simulink model "modello"  (R2019b)
settings: Solver=ode3  StartTime=0.0  StopTime=Tend  FixedStep=Ts  RelTol=1e-3  EnableMultiTasking=on
undefined symbols (not defined in the file): cart_width, masses, nq, q0, q_cart, qp0, qp_cart, qref0, T, tt, xf, xi, xpf, xpi
settings Model: TunableVars=q0,qp0,qref0  TunableVarsStorageClass=Auto,Auto,Auto  TunableVarsTypeQualifier=,,  Creator=danilo  LastModifiedBy=bhisma
settings DataIOCC: LimitDataPoints=on  SaveFormat=Array  ReturnWorkspaceOutputs=off
settings OptimizationCC: DefaultParameterBehavior=Inlined  LifeSpan=inf
settings DebuggingCC: SolverPrmCheckMsg=warning  SFUnexpectedBacktrackingDiag=warning  SFNoUnconditionalDefaultTransitionDiag=warning  SFExecutionAtInitializationDiag=none  ArithmeticOperatorsInVariantConditions=warning
settings HardwareCC: ProdBitPerPointer=32  ProdBitPerSizeT=32  ProdBitPerPtrDiffT=32  ProdLargestAtomicFloat=None  ProdIntDivRoundTo=Undefined  ProdEndianess=Unspecified  ProdWordSize=32  ProdHWDeviceType=32-bit Generic  TargetBitPerLong=64  TargetBitPerPointer=64  TargetBitPerSizeT=64  TargetBitPerPtrDiffT=64  TargetLongLongMode=on  TargetIntDivRoundTo=Zero  TargetEndianess=LittleEndian  TargetWordSize=64  TargetHWDeviceType=MATLAB Host  ProdEqTarget=off
settings ModelReferenceCC: PropagateSignalLabelsOutOfModel=off
settings SFSimCC: SimUseLocalCustomCode=off  CustomCodeUndefinedFunction=UseInterfaceOnly
settings RTWCC: Description=Rapid Simulation Target  SystemTargetFile=rsim.tlc  TemplateMakefile=rsim_default_tmf  RTWUseLocalCustomCode=off  BuildConfiguration=Faster Runs
settings CodeAppCC: StateflowObjectComments=on  MATLABSourceComments=on
settings RSimTargetCC: PreserveStateflowLocalDataDimensions=off
settings ConfigComp: CovMetricSettings=dw  CovHtmlReporting=on  CovSaveCumulativeToWorkspaceVar=on  CovSaveSingleToWorkspaceVar=on  CovExternalEMLEnable=off  CovSFcnEnable=off

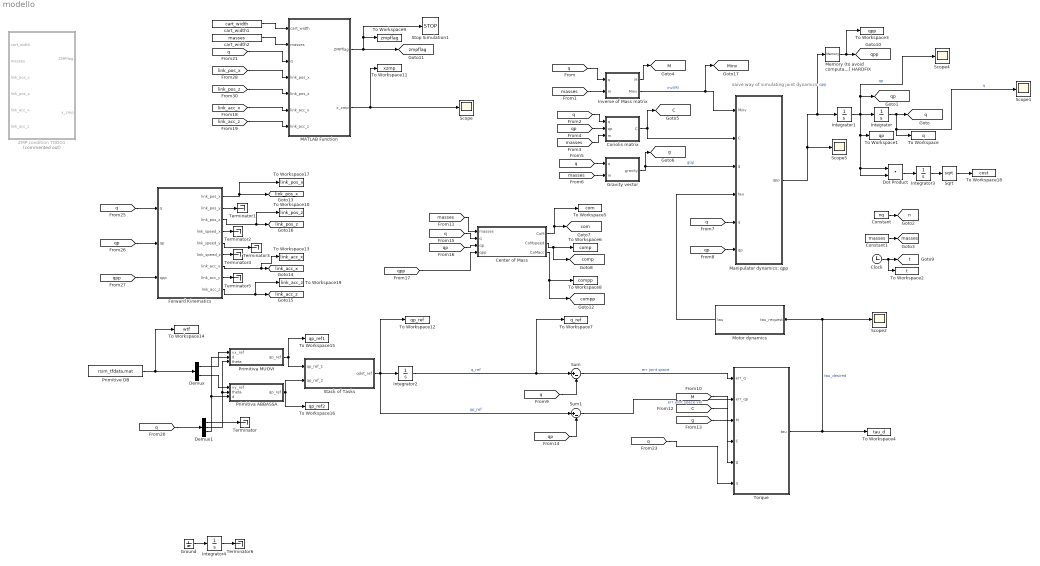
== system modello ==
  note: naive way of simulating joint dynamics
  Center of Mass : MATLAB Function  TreatAsAtomicUnit=on
  Clock : Clock
  Constant : Constant  Value=nq
  Constant1 : Constant  Value=masses
  Coriolis matrix : MATLAB Function  TreatAsAtomicUnit=on
  Demux : Demux  Outputs=2
  Demux1 : Demux  Outputs=3
  Dot Product : DotProduct  InputSameDT=on  OutDataTypeStr=Inherit: Inherit via internal rule
  Forward Kinematics : MATLAB Function  TreatAsAtomicUnit=on
  Gravity vector : MATLAB Function  TreatAsAtomicUnit=on
  Ground : Ground
  Integrator : Integrator  InitialCondition=q0
  Integrator1 : Integrator  InitialCondition=qp0
  Integrator2 : Integrator  InitialCondition=qref0
  Integrator3 : Integrator
  Integrator4 : Integrator  InitialCondition=qref0
  Inverse of Mass matrix : MATLAB Function  TreatAsAtomicUnit=on
  MATLAB Function : MATLAB Function  TreatAsAtomicUnit=on
  Manipulator dynamics: qpp : MATLAB Function  TreatAsAtomicUnit=on
  Memory (to avoid computation of qpp at time 0) HARDFIX : Memory
  Motor dynamics : MATLAB Function  TreatAsAtomicUnit=on
  Primitiva ABBASSA : Subsystem
  Primitiva MUOVI : Subsystem
  Primitive DB : FromFile  FileName=rsim_tfdata.mat  SampleTime=0  ExtrapolationBeforeFirstDataPoint=Hold first value  ExtrapolationAfterLastDataPoint=Hold last value
  Scope{,1..2,4..5} (5 alike) : Scope
  Sqrt : Sqrt  SaturateOnIntegerOverflow=on
  Stack of Tasks : MATLAB Function  TreatAsAtomicUnit=on
  Stop Simulation1 : Stop
  Sum : Sum  Inputs=|+-
  Sum1 : Sum  Inputs=|+-
  Terminator{,1..6} (7 alike) : Terminator
  To Workspace : ToWorkspace  VariableName=q  SampleTime=-1
  To Workspace1 : ToWorkspace  VariableName=qp  SampleTime=-1
  To Workspace10 : ToWorkspace  VariableName=link_pos_z  SampleTime=-1
  To Workspace11 : ToWorkspace  VariableName=xzmp  SampleTime=-1
  To Workspace12 : ToWorkspace  VariableName=qp_ref  SampleTime=-1
  To Workspace13 : ToWorkspace  VariableName=link_acc_x  SampleTime=-1
  To Workspace14 : ToWorkspace  VariableName=wtf  SampleTime=-1
  To Workspace15 : ToWorkspace  VariableName=qp_ref1  SampleTime=-1
  To Workspace16 : ToWorkspace  VariableName=qp_ref2  SampleTime=-1
  To Workspace17 : ToWorkspace  VariableName=link_pos_x  SampleTime=-1
  To Workspace18 : ToWorkspace  VariableName=cost  SampleTime=-1
  To Workspace19 : ToWorkspace  VariableName=link_acc_z  SampleTime=-1
  To Workspace2 : ToWorkspace  VariableName=t  SampleTime=-1
  To Workspace3 : ToWorkspace  VariableName=qpp  SampleTime=-1
  To Workspace4 : ToWorkspace  VariableName=tau_d  SampleTime=-1
  To Workspace5 : ToWorkspace  VariableName=com  SampleTime=-1
  To Workspace6 : ToWorkspace  VariableName=comp  SampleTime=-1
  To Workspace7 : ToWorkspace  VariableName=q_ref  SampleTime=-1
  To Workspace8 : ToWorkspace  VariableName=compp  SampleTime=-1
  To Workspace9 : ToWorkspace  VariableName=zmpflag  SampleTime=-1
  Torque : MATLAB Function  TreatAsAtomicUnit=on
  ZMP condition TODO1 : MATLAB Function  Commented=on  TreatAsAtomicUnit=on
  cart_width1 : Constant  Value=cart_width
  cart_width2 : Constant  Value=masses
  tag scope: C=global, M=global, Minv=global, com=global, comp=global, compp=global, g=global, link_acc_x=global, link_acc_z=global, link_pos_x=global, link_pos_z=global, masses=global, n=global, q=global, qp=global, qpp=global, t=global, zmpflag=global
  wires:
  Integrator1/1 -> Dot Product/2, Dot Product/1, To Workspace1/1, Scope4/1, [qp], Integrator/1  "qp"
  Integrator/1 -> Scope1/1, To Workspace/1, [q]  "q"
  [q] -> Inverse of Mass matrix/1(q)
  Inverse of Mass matrix/2(Minv) -> [Minv], Manipulator dynamics: qpp/1(Minv)  "inv(M)"
  Manipulator dynamics: qpp/1(qpp) -> Scope5/1, Integrator1/1, Memory (to avoid computation of qpp at time 0) HARDFIX/1  "qpp"
  Gravity vector/1(gravity) -> [g], Manipulator dynamics: qpp/3(g)  "g(q)"
  Coriolis matrix/1(C) -> [C], Manipulator dynamics: qpp/2(C)
  Constant/1 -> [n]
  [qp] -> Coriolis matrix/2(qp)
  [q] -> Coriolis matrix/1(q)
  [q] -> Gravity vector/1(q)
  [masses] -> Gravity vector/2(m)
  Torque/1(tau) -> Motor dynamics/1(tau_request), Scope2/1, To Workspace4/1  "tau_desired"
  [q] -> Manipulator dynamics: qpp/5(q)
  [qp] -> Manipulator dynamics: qpp/6(qp)
  Constant1/1 -> [masses]
  [masses] -> Inverse of Mass matrix/2(m)
  [masses] -> Coriolis matrix/3(m)
  Clock/1 -> [t], To Workspace2/1
  Inverse of Mass matrix/1(M) -> [M]
  [M] -> Torque/3(M)
  [C] -> Torque/4(C)
  [g] -> Torque/5(g)
  Motor dynamics/1(tau) -> Manipulator dynamics: qpp/4(tau)
  [masses] -> Center of Mass/1(masses)
  [q] -> Center of Mass/2(q)
  Center of Mass/1(CoM) -> To Workspace5/1, [com]
  [qp] -> Center of Mass/3(qp)
  Center of Mass/2(CoMspeed) -> To Workspace6/1, [comp]
  Sum1/1 -> Torque/2(err_qp)  "err joint space vel"
  [qp] -> Sum1/2
  Stack of Tasks/1(qdot_ref) -> To Workspace12/1, Sum1/1, Integrator2/1  "qp_ref"
  Sum/1 -> Torque/1(err_q)  "err joint space"
  [q] -> Sum/2
  Integrator2/1 -> To Workspace7/1, Sum/1  "q_ref"
  Primitiva MUOVI/1(qp_ref) -> Stack of Tasks/1(qp_ref_1), To Workspace15/1
  Demux/1 -> Primitiva MUOVI/1(vx_ref)
  Demux/2 -> Primitiva ABBASSA/1(vy_ref)
  Primitiva ABBASSA/1(qp_ref) -> Stack of Tasks/2(qp_ref_2), To Workspace16/1
  [q] -> Demux1/1
  Demux1/2 -> Primitiva MUOVI/3(theta), Primitiva ABBASSA/2("theta ")
  Demux1/3 -> Primitiva MUOVI/2(d), Primitiva ABBASSA/3("d ")
  MATLAB Function/1(ZMPflag) -> [zmpflag], To Workspace9/1, Stop Simulation1/1
  MATLAB Function/2(x_zmp) -> To Workspace11/1, Scope/1
  Center of Mass/3(CoMacc) -> [compp], To Workspace8/1
  Demux1/1 -> Terminator/1
  [qpp] -> Center of Mass/4(qpp)
  Memory (to avoid computation of qpp at time 0) HARDFIX/1 -> To Workspace3/1, [qpp]
  Primitive DB/1 -> To Workspace14/1, Demux/1
  [q] -> Forward Kinematics/1(q)
  [qp] -> Forward Kinematics/2(qp)
  [qpp] -> Forward Kinematics/3(qpp)
  Forward Kinematics/1(link_pos_x) -> To Workspace17/1, [link_pos_x]
  Forward Kinematics/2(link_pos_y) -> Terminator1/1
  Forward Kinematics/3(link_pos_z) -> [link_pos_z], To Workspace10/1
  Forward Kinematics/4(link_speed_x) -> Terminator2/1
  Forward Kinematics/6(link_speed_z) -> Terminator4/1
  Forward Kinematics/5(link_speed_y) -> Terminator3/1
  Forward Kinematics/8(link_acc_y) -> Terminator5/1
  Forward Kinematics/9(link_acc_z) -> To Workspace19/1, [link_acc_z]
  Forward Kinematics/7(link_acc_x) -> To Workspace13/1, [link_acc_x]
  cart_width1/1 -> MATLAB Function/1(cart_width)
  [q] -> MATLAB Function/3(q)
  [link_acc_x] -> MATLAB Function/6(link_acc_x)
  [link_acc_z] -> MATLAB Function/7(link_acc_z)
  [link_pos_z] -> MATLAB Function/5(link_pos_z)
  [link_pos_x] -> MATLAB Function/4(link_pos_x)
  cart_width2/1 -> MATLAB Function/2(masses)
  Dot Product/1 -> Integrator3/1
  Integrator3/1 -> Sqrt/1
  Sqrt/1 -> To Workspace18/1
  [q] -> Torque/6(q)
  Ground/1 -> Integrator4/1
  Integrator4/1 -> Terminator6/1

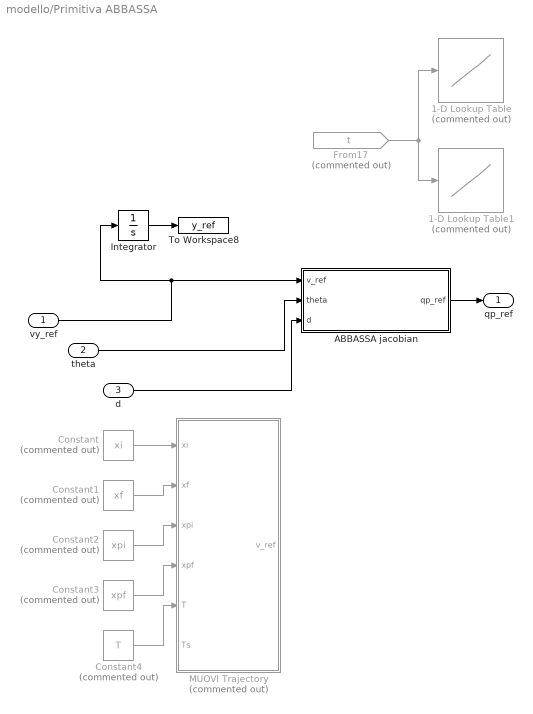
== system modello/Primitiva ABBASSA ==
  vy_ref : Inport
  "theta " : Inport  Port=2
  "d " : Inport  Port=3
  1-D Lookup Table : Lookup_n-D  Commented=on  NumberOfTableDimensions=1  BreakpointsForDimension1=tt  Table=q_cart  ExtrapMethod=Clip  UseLastTableValue=on  InternalRulePriority=Speed  RndMeth=Simplest  InputSameDT=on
  1-D Lookup Table1 : Lookup_n-D  Commented=on  NumberOfTableDimensions=1  BreakpointsForDimension1=tt  Table=qp_cart  ExtrapMethod=Clip  InternalRulePriority=Speed  RndMeth=Simplest  InputSameDT=on
  ABBASSA jacobian : MATLAB Function  TreatAsAtomicUnit=on
  Constant : Constant  Commented=on  Value=xi
  Constant1 : Constant  Commented=on  Value=xf
  Constant2 : Constant  Commented=on  Value=xpi
  Constant3 : Constant  Commented=on  Value=xpf
  Constant4 : Constant  Commented=on  Value=T
  From17 : From  Commented=on  GotoTag=t  TagVisibility=global
  Integrator : Integrator
  MUOVI Trajectory : MATLAB Function  Commented=on  TreatAsAtomicUnit=on
  To Workspace8 : ToWorkspace  VariableName=y_ref  SampleTime=-1
  qp_ref : Outport
  wires:
  ABBASSA jacobian/1(qp_ref) -> qp_ref/1
  From17/1 -> 1-D Lookup Table1/1, 1-D Lookup Table/1
  Integrator/1 -> To Workspace8/1
  Constant/1 -> MUOVI Trajectory/1(xi)
  Constant1/1 -> MUOVI Trajectory/2(xf)
  Constant2/1 -> MUOVI Trajectory/3(xpi)
  Constant3/1 -> MUOVI Trajectory/4(xpf)
  Constant4/1 -> MUOVI Trajectory/5(T)
  "theta "/1 -> ABBASSA jacobian/2(theta)
  "d "/1 -> ABBASSA jacobian/3(d)
  vy_ref/1 -> ABBASSA jacobian/1(v_ref), Integrator/1

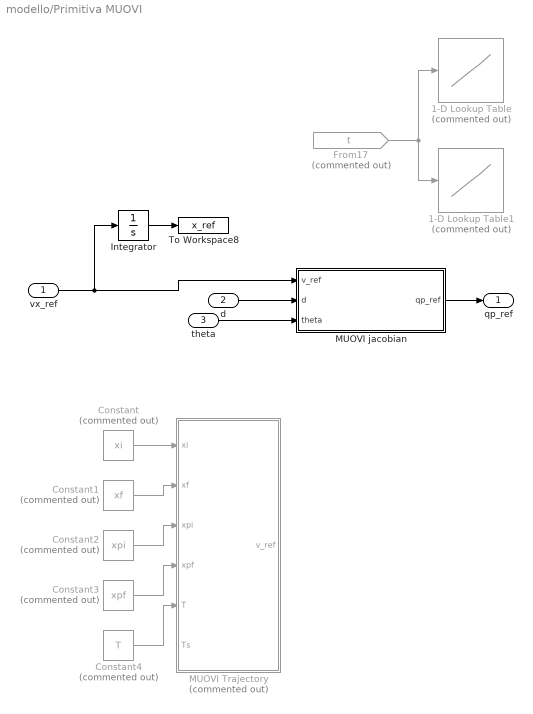
== system modello/Primitiva MUOVI ==
  vx_ref : Inport
  d : Inport  Port=2
  theta : Inport  Port=3
  1-D Lookup Table : Lookup_n-D  Commented=on  NumberOfTableDimensions=1  BreakpointsForDimension1=tt  Table=q_cart  ExtrapMethod=Clip  UseLastTableValue=on  InternalRulePriority=Speed  RndMeth=Simplest  InputSameDT=on
  1-D Lookup Table1 : Lookup_n-D  Commented=on  NumberOfTableDimensions=1  BreakpointsForDimension1=tt  Table=qp_cart  ExtrapMethod=Clip  InternalRulePriority=Speed  RndMeth=Simplest  InputSameDT=on
  Constant : Constant  Commented=on  Value=xi
  Constant1 : Constant  Commented=on  Value=xf
  Constant2 : Constant  Commented=on  Value=xpi
  Constant3 : Constant  Commented=on  Value=xpf
  Constant4 : Constant  Commented=on  Value=T
  From17 : From  Commented=on  GotoTag=t  TagVisibility=global
  Integrator : Integrator
  MUOVI Trajectory : MATLAB Function  Commented=on  TreatAsAtomicUnit=on
  MUOVI jacobian : MATLAB Function  TreatAsAtomicUnit=on
  To Workspace8 : ToWorkspace  VariableName=x_ref  SampleTime=-1
  qp_ref : Outport
  wires:
  MUOVI jacobian/1(qp_ref) -> qp_ref/1
  From17/1 -> 1-D Lookup Table1/1, 1-D Lookup Table/1
  Integrator/1 -> To Workspace8/1
  Constant/1 -> MUOVI Trajectory/1(xi)
  Constant1/1 -> MUOVI Trajectory/2(xf)
  Constant2/1 -> MUOVI Trajectory/3(xpi)
  Constant3/1 -> MUOVI Trajectory/4(xpf)
  Constant4/1 -> MUOVI Trajectory/5(T)
  d/1 -> MUOVI jacobian/2(d)
  theta/1 -> MUOVI jacobian/3(theta)
  vx_ref/1 -> Integrator/1, MUOVI jacobian/1(v_ref)

== matlab function modello/Coriolis matrix ==
  data: q input; qp input; C output; m input
function C = fcn(q,qp,m)
%#codegen

% C = [0,(-1).*m(3).*(cos(q(2)).*q(3).*qp(2)+sin(q(2)).* ...
%   qp(3)),(-1).*m(3).*sin(q(2)).*qp(2); ...
%   0,m(3).*q(3).*qp(3),m(3).*q(3).*qp(2); ...
%   0,(-1).*m(3).*q(3).*qp(2),0];
%% calcolata a mano da lagrangiana
C = [-2.*m(3).*sin(q(2)).*qp(3).*qp(2)-m(3).*q(3).*cos(q(2)).*qp(2)^2;
    2.*m(3).*q(3).*qp(3).*qp(2)-m(3).*sin(q(2)).*qp(1).*qp(3)-m(3).*q(3).*cos(q(2)).*qp(1).*qp(2);
    -m(3).*sin(q(2)).*qp(1).*qp(2)];

== matlab function modello/Inverse of Mass matrix ==
  data: M output; q input; Minv output; m input
function [M,Minv] = fcn(q,m)
%#codegen

% M inversa
Minv = [m(1).^(-1),m(1).^(-1).*q(3).^(-1).*sin(q(2)),(-1).*m(1).^(-1).*cos( ...
  q(2));m(1).^(-1).*q(3).^(-1).*sin(q(2)),m(1).^(-1).*m(3).^(-1).*(m(1)+ ...
  m(3)+(-1).*m(3).*cos(q(2)).^2).*q(3).^(-2),(-1).*m(1).^(-1).*cos(q(2) ...
  ).*q(3).^(-1).*sin(q(2));(-1).*m(1).^(-1).*cos(q(2)),(-1).*m(1).^( ...
  -1).*cos(q(2)).*q(3).^(-1).*sin(q(2)),m(1).^(-1).*m(3).^(-1).*(m(1)+ ...
  m(3)+(-1).*m(3).*sin(q(2)).^2)];

% M non invertita
M = [m(1)+m(3),(-1).*m(3).*q(3).*sin(q(2)),m(3).*cos(q(2));(-1).*m(3).*q(3) ...
   .*sin(q(2)),m(3).*q(3).^2,0;m(3).*cos(q(2)),0,m(3)];

== matlab function modello/Gravity vector ==
  data: q input; gravity output; m input
function gravity = fcn(q,m)
%#codegen
g = 9.81;
% gravity = [0,0,0];
%% calcolato a mano da lagrangiana
gravity = [0;-m(3).*g.*q(3).*cos(q(2));
    m(3).*g.*sin(q(2))];

== matlab function modello/Torque ==
  data: err_q input; err_qp input; tau output; M input; C input; g input; q input
function tau  = fcn(err_q,err_qp,M,C,g,q)
%#codegen
%% calculate control for under-actuated system
err_pos = err_q;
err_vel = err_qp;
% B = [1 0 0;
%     0 0 0;
%     0 0 1];
theta_eq = pi/2;
delta_state = [q(1);theta_eq;q(3)] - q;
% delta_state = zeros(6,1);
% % delta_state = [0;theta_eq;1] - q(:);
% grav = 9.81;
% gpart = [0, 0, 0;
%     0, m(3).*grav.*q(3).*sin(theta_eq), -m(3).*grav.*cos(theta_eq);
%     0, m(3).*grav.*cos(theta_eq), 0];
% % Cpart = [-2.*m(3).*sin(q(2)).*qp(3).*qp(2)-m(3).*q(3).*cos(q(2)).*qp(2)^2;
% %     2.*m(3).*q(3).*qp(3).*qp(2)-m(3).*sin(q(2)).*qp(1).*qp(3)-m(3).*q(3).*cos(q(2)).*qp(1).*qp(2);
% %     -m(3).*sin(q(2)).*qp(1).*qp(2)];
% Cpart = zeros(3,3);
% Alin = [zeros(3,3), eye(3);
%     -Minv*gpart, -Minv*Cpart];
% Blin = [zeros(3,3); Minv*B];
% Q = eye(6);
% R = diag([1 100000 1]);
% K = zeros(3,3);
% % P = lyap(Alin,Q);
% % K = -inv(R)*P*B;%lqr(Alin,Blin,Q,R);
% 
% delta_state = [[0;theta_eq;1] - q(:); -qp-[0;0;0]];
% % Kgain = [ 1.0000   -0.3876    0.0000   20.0230   -8.8656    0.0000;
% %          0         0         0         0         0         0;
% %     0.0000    0.0000    1.0000    0.0000   -0.0000   14.1774];
% Kgain = [316.2278  422.8423    0.0000  503.7380   86.0196   -0.0000;
%          0         0         0         0         0         0;
%    -0.0000   -0.0000  316.2278   -0.0000    0.0000  404.0366];
% Kgain = [31.6228    2.9829    0.0000  116.9117  -22.4599   -0.0000;
%          0         0         0         0         0         0;
%    -0.0000   -0.0000   31.6228   -0.0000    0.0000   85.5836];
% Kgain = 1.0e+03 *[
%     0.4895    3.1493    0.0023    0.9381    0.3620    0.0005;
%     0.0670    0.2088    1.4997    0.0854   -0.0591    0.7999];
% S = [1 0;
%     0 0;
%     0 1];
% tau_eq = [0;
%     981];
% tau = S*(Kgain*delta_state(:) + tau_eq);
% 
% return
%% calculate control for fully-actuated system
tau = zeros(3,1);
% tau(1) = 10;
% tau(3) = 10;

% qref = [1;0;2];
compensate = g+C;
% u = eye(3)*err_q + eye(3)*err_qp;
KP_cart = 100*eye(2);
KP_pend = 10000;
KP = blkdiag(KP_cart,KP_pend);
KD_cart = 10*eye(2);
KD_pend = 100;
KD = blkdiag(KD_cart,KD_pend);
u = KP*err_q + KD*err_qp;
% u =  KD*err_qp;
control = M*(u);
tau = compensate + control;
% tau(2)=0;

== matlab function modello/Manipulator dynamics: qpp ==
  data: Minv input; C input; g input; tau input; q input; qp input; qpp output
function qpp = fcn(Minv,C,g, tau,q,qp)
%#codegen
g = g(:); % column
% qpp = -Minv*(C*qp+g-tau);
%% da lagrangiana
qpp = -Minv*(C+g-tau);

== matlab function modello/Motor dynamics ==
  data: tau_request input; tau output
function tau = fcn(tau_request)
%#codegen

% here we could insert the walkman
% actuator dynamics
tau = tau_request;

== matlab function modello/Forward Kinematics ==
  data: link_pos_x output; q input; qp input; link_pos_y output; qpp input; link_pos_z output; link_speed_x output; link_speed_y output; link_speed_z output; link_acc_x output; link_acc_y output; link_acc_z output
function [link_pos_x,link_pos_y,link_pos_z,link_speed_x,link_speed_y,link_speed_z,link_acc_x,link_acc_y,link_acc_z] = fcn(q,qp,qpp)
%#codegen
% q = [cart position, pendulum angle, pendulum length];
% conventions used here for cartesian axes:
% first  dimension (row) is X (longitudinal)
% second dimension (row) is Y (   lateral  )
% third  dimension (row) is Z (   height   )
link_pos = [q(1), q(1), q(1)+q(3)*cos(q(2));    % X
            0   ,    0, 0;                      % Y
            0   ,    0, q(1)+q(3)*sin(q(2))];   % Z

pxp = qp(1) + qp(3).*cos(q(2)) - q(3).*sin(q(2))*qp(2);
pzp = qp(1) + qp(3).*sin(q(2)) + q(3).*cos(q(2))*qp(2);

link_speed = [qp(1), qp(1), pxp;
                0  ,     0,   0;
                0  ,     0, pzp];

pxpp = qpp(1) + qpp(3).*cos(q(2)) - 2*qp(3).*sin(q(2))*qp(2) - q(3).*cos(q(2))*qp(2)^2 - q(3).*sin(q(2))*qpp(2);
pzpp = qpp(1) + qpp(3).*sin(q(2)) + 2*qp(3).*cos(q(2))*qp(2) - q(3).*sin(q(2))*qp(2)^2 + q(3).*cos(q(2))*qpp(2);

link_acc = [qpp(1), qpp(1), pxpp;
                 0,      0,    0;
                 0,      0, pzpp];
             
% link_pos_x = link_pos(:,1);
% link_pos_y = link_pos(:,2);
% link_pos_z = link_pos(:,3);
% link_speed_x = link_speed(:,1);
% link_speed_y = link_speed(:,2);
% link_speed_z = link_speed(:,3);
% link_acc_x = link_acc(:,1);
% link_acc_y = link_acc(:,2);
% link_acc_z = link_acc(:,3);
link_pos_x = link_pos(1,:);
link_pos_y = link_pos(2,:);
link_pos_z = link_pos(3,:);
link_speed_x = link_speed(1,:);
link_speed_y = link_speed(2,:);
link_speed_z = link_speed(3,:);
link_acc_x = link_acc(1,:);
link_acc_y = link_acc(2,:);
link_acc_z = link_acc(3,:);

== matlab function modello/Primitiva MUOVI/MUOVI jacobian ==
  data: qp_ref output; v_ref input; d input; theta input
function qp_ref  = fcn(v_ref,d,theta)
%#codegen
coder.extrinsic('disp');
coder.extrinsic('num2str');
% jacobian for moving the cart CoM
%J = [1 -d*sin(theta) cos(theta)];
J = [1 0 0];
qp_ref = pinv(J)*v_ref;

== matlab function modello/Stack of Tasks ==
  data: qdot_ref output; qp_ref_1 input; qp_ref_2 input
function qdot_ref = fcn(qp_ref_1,qp_ref_2)
%#codegen

qdot_ref =qp_ref_1 + qp_ref_2;

% qdot_ref =qp_ref_1;

== matlab function modello/Primitiva MUOVI/MUOVI Trajectory ==
  data: v_ref output; xi input; xf input; xpi input; xpf input; T input; Ts input
function v_ref  = fcn(xi,xf,xpi,xpf,T,Ts)
%#codegen
qp_ref = pinv(J)*v_ref;
[a1 a2 a3 a4 a5 a6]=createTraj5(rand,2,0,0,0,0,3,4);
a1 = rand;
vref = 

%%
[a5,a4,a3,a2,a1,a0] = createTraj5(xi,xf,xpi,xpf,0,0,0,T);
coeff=[a5,a4,a3,a2,a1,a0];
coeffp=polyder(coeff);
tt=T(1):Ts:T(2);
% x_cart = polyval(coeff,tt-T(1));
v_cart = polyval(coeffp,tt-T(1));
v_ref = v_cart;

== matlab function modello/Center of Mass ==
  data: masses input; CoM output; q input; qp input; CoMspeed output; qpp input; CoMacc output
function [CoM,CoMspeed,CoMacc] = fcn(masses,q,qp,qpp)
%#codegen
% q = [cart position, pendulum angle, pendulum length];
px = q(1) + q(3).*cos(q(2));
py = q(3).*sin(q(2));

% positions = [q(1), q(2), px];
% CoM = dot(masses,positions)/sum(masses);
% three dimensional CoM calculation
positions = [q(1), q(1), px;
            0, 0, 0;
            0, 0, py];
% CoM_x = dot(masses,positions(:,1))/sum(masses);
% CoM_y = dot(masses,positions(:,2))/sum(masses);
% CoM_z = dot(masses,positions(:,3))/sum(masses);
CoM_x = dot(masses,positions(1,:))/sum(masses);
CoM_y = dot(masses,positions(2,:))/sum(masses);
CoM_z = dot(masses,positions(3,:))/sum(masses);
CoM = [CoM_x; CoM_y; CoM_z];

% center of mass velocity
% positionsdd = [qp(1), qp(2), qp(3)];
% CoMspeed = dot(masses,positionsdd)/sum(masses);
pxp = qp(1) + qp(3).*cos(q(2)) - q(3).*sin(q(2))*qp(2);
pyp = qp(3).*sin(q(2)) + q(3).*cos(q(2))*qp(2);

positionsd = [qp(1), qp(1), pxp;
                0, 0, 0;
                0, 0, pyp];
CoMspeed_x = dot(masses,positionsd(1,:))/sum(masses);
CoMspeed_y = dot(masses,positionsd(2,:))/sum(masses);
CoMspeed_z = dot(masses,positionsd(3,:))/sum(masses);
CoMspeed = [CoMspeed_x;CoMspeed_y;CoMspeed_z];

% center of mass acceleration
% positionsdd = [qpp(1), qpp(2), qpp(3)];
% CoMaccX = dot(masses,positionsdd)/sum(masses);
% CoMaccY = 0;
% CoMaccZ = dot(masses,positionsdd)/sum(masses);
pxpp = qpp(1) + qpp(3).*cos(q(2)) - 2*qp(3).*sin(q(2))*qp(2) - q(3).*cos(q(2))*qp(2)^2 - q(3).*sin(q(2))*qpp(2);
pypp = + qpp(3).*sin(q(2)) + 2*qp(3).*cos(q(2))*qp(2) - q(3).*sin(q(2))*qp(2)^2 + q(3).*cos(q(2))*qpp(2);
positionsdd = [qpp(1), qpp(1), pxpp;
                0, 0, 0;
                0, 0, pypp];

CoMaccX = dot(masses,positionsdd(1,:))/sum(masses);
CoMaccY = dot(masses,positionsdd(2,:))/sum(masses);
CoMaccZ = dot(masses,positionsdd(3,:))/sum(masses);
CoMacc = [CoMaccX;CoMaccY;CoMaccZ];

== matlab function modello/Primitiva ABBASSA/MUOVI Trajectory ==
  data: v_ref output; xi input; xf input; xpi input; xpf input; T input; Ts input
function v_ref  = fcn(xi,xf,xpi,xpf,T,Ts)
%#codegen
qp_ref = pinv(J)*v_ref;
[a1 a2 a3 a4 a5 a6]=createTraj5(rand,2,0,0,0,0,3,4);
a1 = rand;
vref = 

%%
[a5,a4,a3,a2,a1,a0] = createTraj5(xi,xf,xpi,xpf,0,0,0,T);
coeff=[a5,a4,a3,a2,a1,a0];
coeffp=polyder(coeff);
tt=T(1):Ts:T(2);
% x_cart = polyval(coeff,tt-T(1));
v_cart = polyval(coeffp,tt-T(1));
v_ref = v_cart;

== matlab function modello/Primitiva ABBASSA/ABBASSA jacobian ==
  data: qp_ref output; v_ref input; theta input; d input
function qp_ref  = fcn(v_ref,theta,d)
%#codegen
coder.extrinsic('disp');
coder.extrinsic('num2str');
% jacobian for moving the cart CoM
J = [0 d*cos(theta) sin(theta)];
qp_ref = pinv(J)*v_ref;

== matlab function modello/MATLAB Function ==
  data: cart_width input; masses input; ZMPflag output; x_zmp output; q input; link_pos_x input; link_pos_z input; link_acc_x input; link_acc_z input
function [ZMPflag,x_zmp]  = fcn(cart_width,masses,q,link_pos_x,link_pos_z,link_acc_x,link_acc_z)
%#codegen

% zmp calculation
g = [0; 0; -9.81];
pxddot = link_acc_x(:);
pzddot = link_acc_z(:);
px = link_pos_x(:);
pz = link_pos_z(:);
gxvec = g(1)*ones(length(pxddot),1);
gzvec = g(3)*ones(length(pzddot),1);
denominator = dot(masses,pzddot+gzvec);
numerator = zeros(3,1);
numerator(1) =   dot(masses,px.*(pzddot+gzvec));
numerator(2) = - dot(masses,pz.*(pxddot+gxvec));
numerator(3) = 0; % no rotational inertias for now
x_zmp = sum(numerator)/denominator;

% calculate ZMP flag for stability check
x_cart = q(1);
X_cart = [x_cart-cart_width/2;x_cart+cart_width/2];
% ZMPflag = isempty(find(x_zmp >= min(X_cart(1)) & x_zmp <= max(X_cart(2)), 1));
ZMPflag = isempty(find(((x_zmp >= min(X_cart(1))) & (x_zmp <= max(X_cart(2)))),1));
% ZMPflag = (x_zmp >= min(X_cart(1)));

== matlab function modello/ZMP condition TODO1 ==
  data: cart_width input; masses input; ZMPflag output; x_zmp output; link_pos_x input; link_pos_z input; link_acc_x input; link_acc_z input
% This function checks for the ZMP condition
% and returns 1 if it is violated (i.e., robot is falling)
% while 0 if the robot is zmp-stable.
function [ZMPflag,x_zmp]  = fcn(cart_width,masses,link_pos_x,link_pos_z,link_acc_x,link_acc_z)
%#codegen

% function [ZMPflag,x_zmp,y_zmp,x_zmp_ct]  = fcn(cart_width,masses,q,qp,qpp,CoM,CoMacc,link_pos,link_speed,link_acc)
% % q = [cart position, pendulum angle, pendulum length];
% x_cart = q(1);
% X_cart = [x_cart-cart_width/2;x_cart+cart_width/2];
% 
% %% true ZMP
% % zmp data
% % Note: for ZMP calculation there is the following
% % convention: z is the vertical axis, on which the
% % gravity occurs
% g = 9.81;
% % coordinates of the mass center of the links
% xcm = [q(1), q(1), q(1) + q(3).*cos(q(2))];
% ycm = [0, 0, 0]; % y here is the 'depth' direction
% zcm = [0, 0, q(3).*sin(q(2))];
% xcm = CoM(1,:);
% ycm = CoM(2,:);
% zcm = CoM(3,:);
% % acceleration of the robot center of mass
% xx = CoMacc(1); 
% yy = CoMacc(2); % not used, left here for generality
% zz = CoMacc(3);
% % acceleration of the links around the x-y axis
% thetaxpp = [0, 0, 0]; % not used, left here for generality
% thetaypp = [0 qp(2) 0*qpp(2)]; % not sure about the third element
% % rotational inertia about the x-y axis
% inx = [0 0 0]; % not used, left here for generality
% iny = [0 1/2*masses(2)*1^2 1/12*masses(3)*q(3)^2]; % radius of  the rotational d.o.f. inertia = 1
% %% zmp denominator (common for both x and y zmp values)
% div = ((zz+g)*sum(masses));
% %% zmp horizontal-value
% x_zmp = g*zz*dot(masses,xcm) - xx*dot(masses,zcm) - dot(iny,thetaypp);
% %
% % div = dot(masses,zcm+g);
% % CoM
% % CoMacc
% % sum_1 = dot(masses.*xcm,-g+
% % x_zmp = g*zz*dot(masses,xcm) - xx*dot(masses,zcm) - dot(iny,thetaypp);
% 
% %
% x_zmp = x_zmp/div;
% % x_zmp = sum(masses)*(-g)*CoM(1)/(sum(masses)*(-g)+CoMacc(3));
% % x_zmp = sum(masses)*(-g)*CoM(1)/(sum(masses)*(-g));
% %% zmp vertical-value
% y_zmp = g*zz*dot(masses,ycm) - xx*dot(masses,zcm) - dot(inx,thetaxpp);
% y_zmp = y_zmp/div;
% 
% % % check if CoM value lies between the extreme values of X_cart vector
% % ZMPflag = isempty(find(CoM >= min(X_cart(1)) & CoM <= max(X_cart(2)), 1));
% % check if ZMP x-value lies between the extreme values of X_cart vector
% ZMPflag = isempty(find(x_zmp >= min(X_cart(1)) & x_zmp <= max(X_cart(2)), 1));
% 
% % x_zmp calculated with the cart-table approximation
% x_com = CoM(1);
% z_com = CoM(3);
% x_zmp_ct = x_com - z_com*zz/g;

%% Huang et al. assuming height of ZMP on the ground is 0 (i.e. on the floor)
g = [0; 0; -9.81];
gz = g(3);
pxddot = link_acc_x;
pzddot = link_acc_z;
px = link_pos_x;
pz = link_pos_z;

denominator = dot(masses,pzddot+gz);
numerator = zeros(3,1);
numerator(1) =   dot(masses,px.*(pzddot+gz));
numerator(2) = - dot(masses,pz.*(pxddot+gz));
numerator(3) = 0; % no rotational inertias for now
x_zmp = sum(numerator)/denominator;
% check if ZMP x-value lies between the extreme values of X_cart vector
x_cart = q(1);
X_cart = [x_cart-cart_width/2;x_cart+cart_width/2];
ZMPflag = isempty(find(x_zmp >= min(X_cart(1)) & x_zmp <= max(X_cart(2)), 1));
